simulink model "ECS3"  (R2019b)
settings: Solver=FixedStepAuto  StartTime=0.0  StopTime=inf  RelTol=1e-3  EnableMultiTasking=on
settings Model: SimulationMode=external  EnablePacing=on  Creator=krist  LastModifiedBy=krist
settings SolverCC: PositivePriorityOrder=on
settings OptimizationCC: EnhancedBackFolding=on  PassReuseOutputArgsAs=Individual arguments  ZeroExternalMemoryAtStartup=off  ZeroInternalMemoryAtStartup=off  MaxStackSize=64  OptimizeBlockOrder=speed  DifferentSizesBufferReuse=on  OptimizationCustomize=off  EfficientTunableParamExpr=on
settings DebuggingCC: ParameterTunabilityLossMsg=error
settings HardwareCC: ProdBitPerPointer=32  ProdBitPerSizeT=32  ProdBitPerPtrDiffT=32  ProdLargestAtomicInteger=Long  ProdLargestAtomicFloat=Double  ProdWordSize=32  ProdLongLongMode=on  ProdHWDeviceType=ARM Compatible->ARM Cortex
settings RTWCC: SystemTargetFile=ert.tlc  HardwareBoard=Raspberry Pi  TLCOptions="-aInlineSetEventsForThisBaseRateFcn=TLC_FALSE -aSuppressMultiTaskScheduler=TLC_FALSE  -aRateBasedStepFcn=0"  TemplateMakefile=ert_default_tmf  GenerateReport=on  Toolchain=GNU GCC Raspberry Pi  BuildConfiguration=Faster Runs  IncludeHyperlinkInReport=on  LaunchReport=on  GenerateTraceInfo=on  GenerateTraceReport=on  GenerateTraceReportSl=on  GenerateTraceReportSf=on  GenerateTraceReportEml=on
settings CodeAppCC: ForceParamTrailComments=on  IgnoreCustomStorageClasses=off  OperatorAnnotations=on  SimulinkDataObjDesc=on  SFDataObjDesc=on  InsertBlockDesc=on
settings ERTTargetCC: SupportVariableSizeSignals=on  ExtMode=on  ExtModeTransport=2  ExtModeStaticAlloc=on  ExtModeMexFile=ext_xcp  ExtModeMexArgs='169.254.0.2' 0 17725  ExtModeIntrfLevel=Level2 - Open

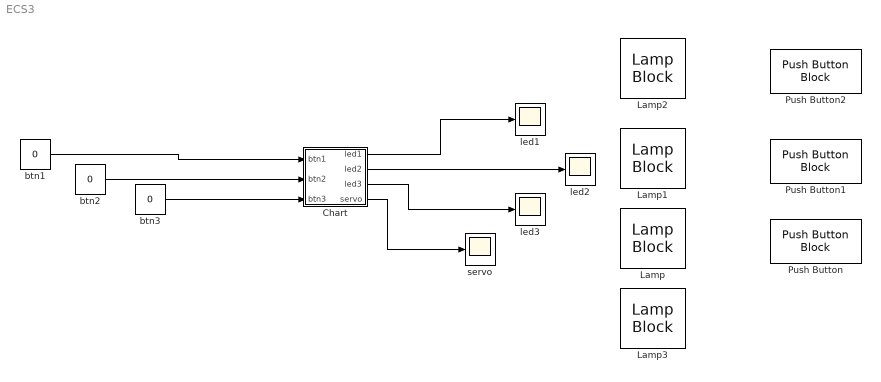
== system ECS3 ==
  Chart : Stateflow chart  BlockKeywords=__PRM__SERIALIZED__DATA__:Stateflow Chart,Stateflow Diagram  TreatAsAtomicUnit=on
  Lamp{,1..3} (4 alike) : LampBlock
  Push Button : PushButtonBlock
  Push Button1 : PushButtonBlock
  Push Button2 : PushButtonBlock
  btn1 : Constant  Value=0
  btn2 : Constant  Value=0
  btn3 : Constant  Value=0
  led1 : Scope
  led2 : Scope
  led3 : Scope
  servo : Scope
  wires:
  btn3/1 -> Chart/3(btn3)
  btn2/1 -> Chart/2(btn2)
  Chart/1(led1) -> led1/1
  Chart/2(led2) -> led2/1
  Chart/3(led3) -> led3/1
  Chart/4(servo) -> servo/1
  btn1/1 -> Chart/1(btn1)

== stateflow chart ECS3/Chart ==
  state Start
    led1=1;
    prevFloor=1;
  state state6b
  state state6a
  state Moving
    led1=0;
    led2=0;
    led3=0;
  state Arrive
    servo=1;
    ms=0;
    prevFloor=floor;
  state Idle
  state state2
  state state3
  state state8
  state state6
  state state7
  (default) -> Start
  Start -> Idle
  state6a -> state6b : after(1,sec){led2=0}
  state6b -> state7 : after(3,sec)
  state6 -> state6a [order 1] : [floor-prevFloor==-2]{led2=1}
  state6 -> state6a [order 2] : [floor-prevFloor==2]{led2=1}
  Idle -> state2 [order 1] : [btn1==1]{floor=1}
  state2 -> state3 [order 1] : [floor>prevFloor]{servo=0.5;}
  Idle -> state2 [order 2] : [btn2==1]{floor=2}
  state3 -> Moving : after(1,sec)
  state7 -> state8 [order 2] : [floor==1]{led1=1}
  state2 -> state3 [order 2] : [floor<prevFloor]{servo=0.9;}
  Idle -> state2 [order 3] : [btn3==1]{floor=3}
  state7 -> state8 [order 1] : [floor==2]{led2=1}
  state8 -> Arrive : after(1,sec)
  state2 -> Idle [order 3]
  state7 -> state8 [order 3] : [floor==3]{led3=1}
  state6 -> state7 [order 3]
  Moving -> state6 : after(3,sec)
  Arrive -> Idle
  data: btn1 input; btn2 input; btn3 input; led1 output; led2 output; led3 output; floor local; servo output; ms local; prevFloor local
